simulink model "NavFilterTestHarness24"  (Simulink 7.9)
settings: Solver=FixedStepDiscrete  StartTime=min(IMUtime)  StopTime=max(IMUtime)  FixedStep=0.001  RelTol=1e-3
undefined symbols (not defined in the file or in its folder): accel, ADSframe, ADStime, angRate, ATTframe, CourseDeg, GndSpd, GPSframe, GPStime, Hgt, IMUframe, IMUtime, LatDeg, LngDeg, MagBiasX, MagBiasY, MagBiasZ, MAGframe, MAGtime, MagX, MagY, MagZ, Pitch, Roll, Veas, VelD, Yaw
libraries: simulink x15
(part 2 of 5)

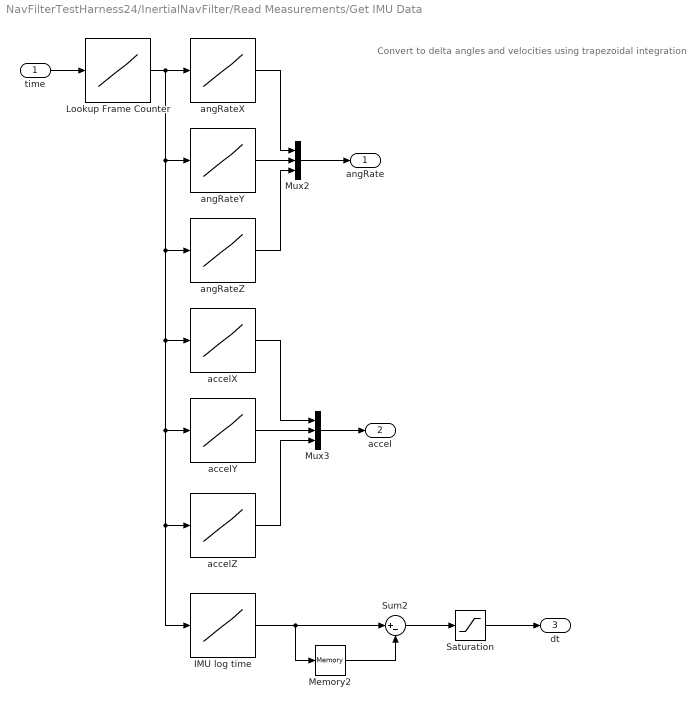
== system NavFilterTestHarness24/InertialNavFilter/Read Measurements/Get IMU Data ==
  note: Convert to delta angles and velocities using trapezoidal integration
  time : Inport
  IMU log time : Lookup_n-D  NumberOfTableDimensions=1  BreakpointsForDimension1=IMUframe  BeginIndexSearchUsingPreviousIndexResult=on  Table=IMUtime  InterpMethod=Flat  DiagnosticForOutOfRangeInput=Error  OutDataTypeStr=single  RndMeth=Simplest  InputSameDT=on
  Lookup Frame Counter : Lookup_n-D  NumberOfTableDimensions=1  BreakpointsForDimension1=IMUtime  BeginIndexSearchUsingPreviousIndexResult=on  Table=IMUframe  InterpMethod=Flat  DiagnosticForOutOfRangeInput=Error  RndMeth=Simplest  InputSameDT=on
  Memory2 : Memory  InheritSampleTime=on
  Mux2 : Mux  Inputs=3
  Mux3 : Mux  Inputs=3
  Saturation : Saturate  UpperLimit=0.04  LowerLimit=0
  Sum2 : Sum  Inputs=|+-  AccumDataTypeStr=single
  accelX : Lookup_n-D  NumberOfTableDimensions=1  BreakpointsForDimension1=IMUframe  BeginIndexSearchUsingPreviousIndexResult=on  Table=accel(:,1)  InterpMethod=Flat  DiagnosticForOutOfRangeInput=Error  OutDataTypeStr=single  RndMeth=Simplest  InputSameDT=on
  accelY : Lookup_n-D  NumberOfTableDimensions=1  BreakpointsForDimension1=IMUframe  BeginIndexSearchUsingPreviousIndexResult=on  Table=accel(:,2)  InterpMethod=Flat  DiagnosticForOutOfRangeInput=Error  OutDataTypeStr=single  RndMeth=Simplest  InputSameDT=on
  accelZ : Lookup_n-D  NumberOfTableDimensions=1  BreakpointsForDimension1=IMUframe  BeginIndexSearchUsingPreviousIndexResult=on  Table=accel(:,3)  InterpMethod=Flat  DiagnosticForOutOfRangeInput=Error  OutDataTypeStr=single  RndMeth=Simplest  InputSameDT=on
  angRateX : Lookup_n-D  NumberOfTableDimensions=1  BreakpointsForDimension1=IMUframe  BeginIndexSearchUsingPreviousIndexResult=on  Table=angRate(:,1)  InterpMethod=Flat  DiagnosticForOutOfRangeInput=Error  OutDataTypeStr=single  RndMeth=Simplest  InputSameDT=on
  angRateY : Lookup_n-D  NumberOfTableDimensions=1  BreakpointsForDimension1=IMUframe  BeginIndexSearchUsingPreviousIndexResult=on  Table=angRate(:,2)  InterpMethod=Flat  DiagnosticForOutOfRangeInput=Error  OutDataTypeStr=single  RndMeth=Simplest  InputSameDT=on
  angRateZ : Lookup_n-D  NumberOfTableDimensions=1  BreakpointsForDimension1=IMUframe  BeginIndexSearchUsingPreviousIndexResult=on  Table=angRate(:,3)  InterpMethod=Flat  DiagnosticForOutOfRangeInput=Error  OutDataTypeStr=single  RndMeth=Simplest  InputSameDT=on
  angRate : Outport  OutDataTypeStr=single
  accel : Outport  Port=2
  dt : Outport  Port=3  OutDataTypeStr=single
  wires:
  accelY/1 -> Mux3/2
  accelX/1 -> Mux3/1
  accelZ/1 -> Mux3/3
  angRateX/1 -> Mux2/1
  angRateY/1 -> Mux2/2
  angRateZ/1 -> Mux2/3
  Lookup Frame Counter/1 -> angRateX/1, angRateY/1, angRateZ/1, accelX/1, accelY/1, accelZ/1, IMU log time/1
  time/1 -> Lookup Frame Counter/1
  IMU log time/1 -> Sum2/1, Memory2/1
  Memory2/1 -> Sum2/2
  Mux2/1 -> angRate/1
  Mux3/1 -> accel/1
  Sum2/1 -> Saturation/1
  Saturation/1 -> dt/1

== system NavFilterTestHarness24/LogData/GetReferenceData/wrapAng to +-pi ==
  In1 : Inport  OutDataTypeStr=single
  If : If  IfExpression=u1 > single(pi)
  If Action Subsystem : Subsystem  TreatAsAtomicUnit=on
  If Action Subsystem1 : Subsystem  TreatAsAtomicUnit=on
  Merge : Merge
  Out1 : Outport  OutDataTypeStr=single
  wires:
  In1/1 -> If Action Subsystem1/1(In1), If Action Subsystem/1(In1), If/1
  If/2 -> If Action Subsystem/Action
  If/1 -> If Action Subsystem1/Action
  If Action Subsystem/1(Out1) -> Merge/1
  If Action Subsystem1/1(Out1) -> Merge/2
  Merge/1 -> Out1/1

== system NavFilterTestHarness24/WatchDog/Get AHRS Data/wrapAng to +-pi ==
  In1 : Inport  OutDataTypeStr=single
  If : If  IfExpression=u1 > single(pi)
  If Action Subsystem : Subsystem  TreatAsAtomicUnit=on
  If Action Subsystem1 : Subsystem  TreatAsAtomicUnit=on
  Merge : Merge
  Out1 : Outport  OutDataTypeStr=single
  wires:
  In1/1 -> If Action Subsystem1/1(In1), If Action Subsystem/1(In1), If/1
  If/2 -> If Action Subsystem/Action
  If/1 -> If Action Subsystem1/Action
  If Action Subsystem/1(Out1) -> Merge/1
  If Action Subsystem1/1(Out1) -> Merge/2
  Merge/1 -> Out1/1

== system NavFilterTestHarness24/InertialNavFilter/CalculateInitialStates/Read AHRS solution/wrapAng to +-pi ==
  In1 : Inport  OutDataTypeStr=single
  If : If  IfExpression=u1 > single(pi)
  If Action Subsystem : Subsystem  TreatAsAtomicUnit=on
  If Action Subsystem1 : Subsystem  TreatAsAtomicUnit=on
  Merge : Merge
  Out1 : Outport  OutDataTypeStr=single
  wires:
  In1/1 -> If Action Subsystem1/1(In1), If Action Subsystem/1(In1), If/1
  If/2 -> If Action Subsystem/Action
  If/1 -> If Action Subsystem1/Action
  If Action Subsystem/1(Out1) -> Merge/1
  If Action Subsystem1/1(Out1) -> Merge/2
  Merge/1 -> Out1/1

== system NavFilterTestHarness24/LogData/GetReferenceData/wrapAng to +-pi/If Action Subsystem ==
  In1 : Inport
  Action Port : ActionPort  ActionType=else
  Out1 : Outport
  wires:
  In1/1 -> Out1/1

== system NavFilterTestHarness24/LogData/GetReferenceData/wrapAng to +-pi/If Action Subsystem1 ==
  In1 : Inport
  Action Port : ActionPort  ActionType=then
  Add : Sum  Inputs=+-
  Constant : Constant  Value=2*pi  OutDataTypeStr=single
  Out1 : Outport
  wires:
  In1/1 -> Add/1
  Add/1 -> Out1/1
  Constant/1 -> Add/2

== system NavFilterTestHarness24/WatchDog/Get AHRS Data/wrapAng to +-pi/If Action Subsystem ==
  In1 : Inport
  Action Port : ActionPort  ActionType=else
  Out1 : Outport
  wires:
  In1/1 -> Out1/1

== system NavFilterTestHarness24/WatchDog/Get AHRS Data/wrapAng to +-pi/If Action Subsystem1 ==
  In1 : Inport
  Action Port : ActionPort  ActionType=then
  Add : Sum  Inputs=+-
  Constant : Constant  Value=2*pi  OutDataTypeStr=single
  Out1 : Outport
  wires:
  In1/1 -> Add/1
  Add/1 -> Out1/1
  Constant/1 -> Add/2

== system NavFilterTestHarness24/InertialNavFilter/CalculateInitialStates/Read AHRS solution/wrapAng to +-pi/If Action Subsystem ==
  In1 : Inport
  Action Port : ActionPort  ActionType=else
  Out1 : Outport
  wires:
  In1/1 -> Out1/1

== system NavFilterTestHarness24/InertialNavFilter/CalculateInitialStates/Read AHRS solution/wrapAng to +-pi/If Action Subsystem1 ==
  In1 : Inport
  Action Port : ActionPort  ActionType=then
  Add : Sum  Inputs=+-
  Constant : Constant  Value=2*pi  OutDataTypeStr=single
  Out1 : Outport
  wires:
  In1/1 -> Add/1
  Add/1 -> Out1/1
  Constant/1 -> Add/2

== matlab function WatchDog/wrapAnglePi ==
  data: angleOut output double; angleIn input double
function angleOut   = wrapAnglePi(angleIn)
%#codegen

if abs(angleIn) <= pi
    angleOut = angleIn;
elseif  angleIn < -pi
    angleOut = angleIn + 2*pi;
elseif angleIn > pi
    angleOut = angleIn - 2*pi;
else
    angleOut = angleIn;
end

end

== matlab function InertialNavFilter/Predict States ==
  data: nextStates output double; correctedDelAng output double; correctedDelVel output double; accNavMag output double; states input double; earthRateNED input double; dAngIMU input double; dVelIMU input double; dtIMU input double
%#codegen
function [nextStates,correctedDelAng,correctedDelVel,accNavMag]  = UpdateStrapdownEquationsNED( ...
    states, ...
    earthRateNED, ...
    dAngIMU, ...
    dVelIMU, ...
    dtIMU)

% define persistent variables for previous delta angle and velocity which
% are required for sculling and coning error corrections
persistent prevDelAng;
if isempty(prevDelAng)
    prevDelAng = single([0;0;0]);
end
persistent Tbn;
if isempty(Tbn)
    Tbn = single(eye(3));
end

gravityNED = [0.0;0.0;9.80665];

% Remove sensor bias errors
correctedDelAng = dAngIMU - states(11:13);
correctedDelVel = dVelIMU - states(14:16);

% Save current measurements
prevDelAng = correctedDelAng;

% Apply corrections for earths rotation rate and coning errors
correctedDelAng   = correctedDelAng - transpose(Tbn)*earthRateNED*dtIMU + 8.333333333333333e-2*cross(prevDelAng , dAngIMU);

% Initialise the updated state vector
nextStates   = states;

% Convert the rotation vector to its equivalent quaternion
rotationMag = sqrt(correctedDelAng(1)^2 + correctedDelAng(2)^2 + correctedDelAng(3)^2);
if rotationMag<1e-12
  deltaQuat = single([1;0;0;0]);
else
  deltaQuat = [cos(0.5*rotationMag); correctedDelAng/rotationMag*sin(0.5*rotationMag)];
end

% Update the quaternions by rotating from the previous attitude through
% the delta angle rotation quaternion
qUpdated = [states(1)*deltaQuat(1)-transpose(states(2:4))*deltaQuat(2:4); states(1)*deltaQuat(2:4) + deltaQuat(1)*states(2:4) + cross(states(2:4),deltaQuat(2:4))];

% Normalise the quaternions and update the quaternion states
quatMag = sqrt(qUpdated(1)^2 + qUpdated(2)^2 + qUpdated(3)^2 + qUpdated(4)^2);
if (quatMag < 1e-16)
    nextStates(1:4) = qUpdated;
else
    nextStates(1:4) = qUpdated / quatMag;
end

% Calculate the body to nav cosine matrix
Tbn = [nextStates(1)^2 + nextStates(2)^2 - nextStates(3)^2 - nextStates(4)^2, 2*(nextStates(2)*nextStates(3) - nextStates(1)*nextStates(4)), 2*(nextStates(2)*nextStates(4) + nextStates(1)*nextStates(3));...
      2*(nextStates(2)*nextStates(3) + nextStates(1)*nextStates(4)), nextStates(1)^2 - nextStates(2)^2 + nextStates(3)^2 - nextStates(4)^2, 2*(nextStates(3)*nextStates(4) - nextStates(1)*nextStates(2));...
      2*(nextStates(2)*nextStates(4)-nextStates(1)*nextStates(3)), 2*(nextStates(3)*nextStates(4) + nextStates(1)*nextStates(2)), nextStates(1)^2 - nextStates(2)^2 - nextStates(3)^2 + nextStates(4)^2];
  
% transform body delta velocities to delta velocities in the nav frame
delVelNav = Tbn * correctedDelVel + gravityNED*dtIMU;

% calculate the magnitude of the nav acceleration (required for GPS
% variance estimation)
accNavMag = sqrt(delVelNav(1)^2 + delVelNav(2)^2 + delVelNav(3)^2) / dtIMU;

% If calculating position save previous velocity
lastVelocity = nextStates(5:7);

% Sum delta velocities to get velocity after removing gravitational skew and correcting for transport rate
nextStates(5:7) = states(5:7) + delVelNav;


% If calculating postions, do a trapezoidal integration for position
nextStates(8:10)     = states(8:10) + 0.5*(nextStates(5:7) + lastVelocity)*dtIMU;

% Copy the remaining states across
nextStates(11:24) = states(11:24);

end
